simulink model "autopilot2f"  (R2017a)
settings: Solver=VariableStepAuto  StartTime=0.0  StopTime=300  RelTol=1e-3
values from neighbouring files (symbols this model uses):
  A = [-0.322     0.052   0.028   -1.12   0.002 ... (first row only)    [run_task_2f.m]
  B = [0; 0; 0; 0; 10]    [run_task_2f.m]
  C = [0 0 0 1 0 ... (first row only)    [run_task_2f.m]
  d = 2*deg2rad    (= 0.0349065850399)    [run_task_2f.m]
  D = zeros(4, 1)    [run_task_2f.m]
  g = 9.81    [auoschmilot.m]    (also in run_task_2f.m)
  k_d_phi = (2*zeta_phi*w_n_phi-a_1)/a_2    [auoschmilot.m]    (also in run_task_2f.m)
  k_i_x = 0.195    [auoschmilot.m]    (also in run_task_2f.m)
  k_p_phi = -5/3    (= -1.66666666667)    [auoschmilot.m]    (also in run_task_2f.m)
  k_p_x = 2*zeta_X*w_n_x*V_g/g    [auoschmilot.m]    (also in run_task_2f.m)
  large_step = 30    [run_task_2f.m]
  V_g = 637/3.6    (= 176.944444444)    [auoschmilot.m]    (also in run_task_2f.m)
libraries: simulink_extras x3
settings Model: Creator=rokru  LastModifiedBy=emilal

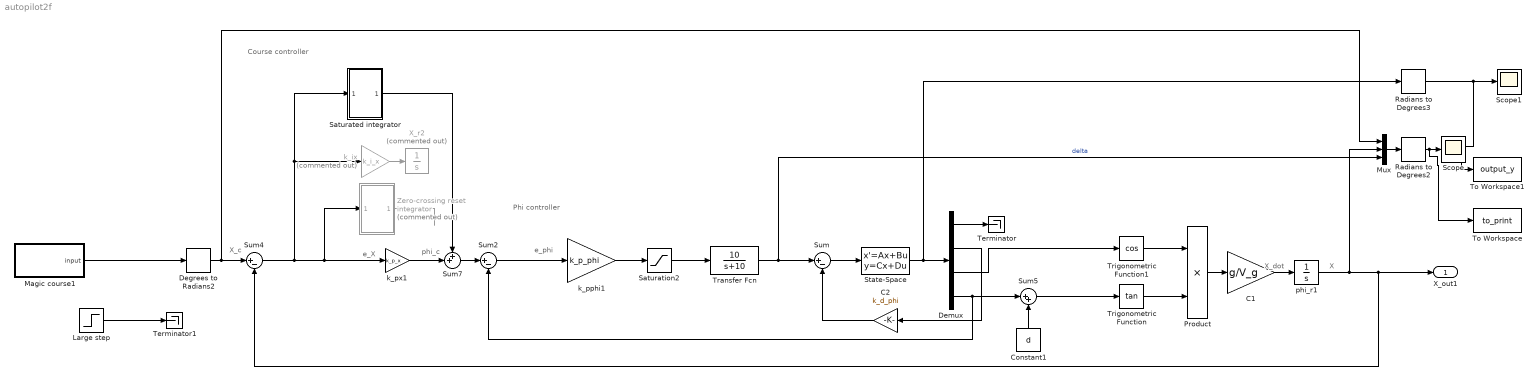
== system autopilot2f ==
  note: X
  note: X_c
  note: X_dot
  note: phi_c
  note: Course controller
  note: e_X
  note: Phi controller
  note: e_phi
  C1 : Gain  Gain=g/V_g
  C2 : Gain  Gain=k_d_phi
  Constant1 : Constant  Value=d
  Degrees to Radians2 : simulink_extras/Transformations/Degrees to Radians
  Demux : Demux
  Large step : Step  Time=50  After=large_step  SampleTime=0
  Magic course1 : Subsystem
  Mux : Mux  Inputs=3
  Product : Product
  Radians to Degrees2 : simulink_extras/Transformations/Radians to Degrees
  Radians to Degrees3 : simulink_extras/Transformations/Radians to Degrees
  Saturated integrator : Subsystem
  Saturation2 : Saturate  UpperLimit=25*deg2rad  LowerLimit=-25*deg2rad
  Scope : Scope
  Scope1 : Scope
  State-Space : StateSpace  A=A  B=B  C=C  D=D  X0=0
  Sum : Sum  Inputs=|+-
  Sum2 : Sum  Inputs=|+-
  Sum4 : Sum  Inputs=|+-
  Sum5 : Sum  Inputs=|++
  Sum7 : Sum  Inputs=++|
  Terminator : Terminator
  Terminator1 : Terminator
  To Workspace : ToWorkspace  VariableName=to_print  SaveFormat=Timeseries  SampleTime=-1
  To Workspace1 : ToWorkspace  VariableName=output_y  SaveFormat=Timeseries  SampleTime=-1
  Transfer Fcn : TransferFcn  Numerator=[10]  Denominator=[1 10]
  Trigonometric Function : Trigonometry  Operator=tan
  Trigonometric Function1 : Trigonometry  Operator=cos
  X_r2 : Integrator  Commented=on
  "Zero-crossing reset integrator " : Subsystem  Commented=on
  k_ix : Gain  Commented=on  Gain=k_i_x
  k_pphi1 : Gain  Gain=k_p_phi
  k_px1 : Gain  Gain=k_p_x
  phi_r1 : Integrator
  X_out1 : Outport
  wires:
  State-Space/1 -> Radians to Degrees3/1, Demux/1
  Trigonometric Function/1 -> Product/2
  C1/1 -> phi_r1/1
  k_px1/1 -> Sum7/2
  Sum4/1 -> Saturated integrator/1(In1), k_ix/1, "Zero-crossing reset integrator "/1(In1), k_px1/1
  Product/1 -> C1/1
  C2/1 -> Sum/2
  Saturation2/1 -> Transfer Fcn/1
  Mux/1 -> Radians to Degrees2/1
  Demux/3 -> Trigonometric Function1/1
  Trigonometric Function1/1 -> Product/1
  Demux/2 -> C2/1
  Demux/4 -> Sum5/1, Sum2/2
  Sum/1 -> State-Space/1
  Constant1/1 -> Sum5/2
  k_pphi1/1 -> Saturation2/1
  Sum7/1 -> Sum2/1
  Sum2/1 -> k_pphi1/1
  Sum5/1 -> Trigonometric Function/1
  Magic course1/1(input) -> Degrees to Radians2/1
  Transfer Fcn/1 -> Mux/3, Sum/1  "delta"
  phi_r1/1 -> Mux/2, X_out1/1, Sum4/2
  Degrees to Radians2/1 -> Mux/1, Sum4/1
  Radians to Degrees3/1 -> To Workspace1/1, Scope1/1
  Radians to Degrees2/1 -> To Workspace/1, Scope/1
  Demux/1 -> Terminator/1
  Large step/1 -> Terminator1/1
  "Zero-crossing reset integrator "/1(Out1) -> ?
  k_ix/1 -> X_r2/1
  Saturated integrator/1(Out1) -> Sum7/1

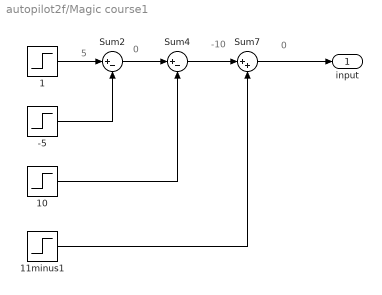
== system autopilot2f/Magic course1 ==
  note: 0
  note: -10
  note: 0
  note: 5
  -5 : Step  Time=100  After=5  SampleTime=0
  1 : Step  Time=10  After=5  SampleTime=0
  10 : Step  Time=150  After=10  SampleTime=0
  11minus1 : Step  Time=200  After=10  SampleTime=0
  Sum2 : Sum  Inputs=|+-
  Sum4 : Sum  Inputs=|+-
  Sum7 : Sum  Inputs=|++
  input : Outport
  wires:
  10/1 -> Sum4/2
  11minus1/1 -> Sum7/2
  -5/1 -> Sum2/2
  Sum7/1 -> input/1
  1/1 -> Sum2/1
  Sum4/1 -> Sum7/1
  Sum2/1 -> Sum4/1

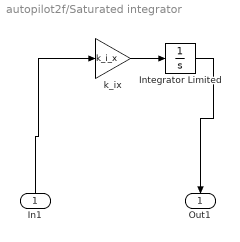
== system autopilot2f/Saturated integrator ==
  In1 : Inport
  Integrator Limited : Integrator  LimitOutput=on  UpperSaturationLimit=0.06  LowerSaturationLimit=-0.06
  k_ix : Gain  Gain=k_i_x
  Out1 : Outport
  wires:
  k_ix/1 -> Integrator Limited/1
  Integrator Limited/1 -> Out1/1
  In1/1 -> k_ix/1

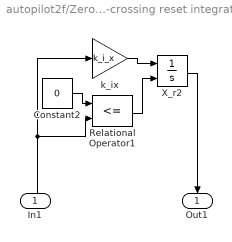
== system autopilot2f/Zero-crossing reset integrator  ==
  In1 : Inport
  Constant2 : Constant  Value=0
  Relational Operator1 : RelationalOperator  Operator=<=  OutDataTypeStr=boolean  RndMeth=Simplest
  X_r2 : Integrator  ExternalReset=level
  k_ix : Gain  Gain=k_i_x
  Out1 : Outport
  wires:
  Constant2/1 -> Relational Operator1/1
  Relational Operator1/1 -> X_r2/2
  k_ix/1 -> X_r2/1
  X_r2/1 -> Out1/1
  In1/1 -> Relational Operator1/2, k_ix/1
